simulink model "astron_hw_test_au50_64k"  (R2021a)
settings: Solver=VariableStepDiscrete  StartTime=0.0  StopTime=2048  RelTol=1e-3
undefined symbols (not defined in the file): d0, d1, d2, d3, FFT, sr, Wideband_FFT
libraries: xbsIndex_r4 x637, casper_library_misc x4, xps_library x1
(part 2 of 14)

== system astron_hw_test_au50_64k/bram_in0 ==
  addr : Inport
  data_in : Inport  Port=2
  we : Inport  Port=3
  Terminator : Terminator
  Terminator1 : Terminator
  Terminator2 : Terminator
  astron_hw_test_au50_64k_bram_in0_addr : xbsIndex_r4/Gateway Out  inherit_from_input=off  hdl_port=on  rows=1  columns=1  UseAsDAC=off  DACChannel='1'  interface=None  automatic_assignment=on  address_offset=hex2dec('00')  intf_name=''  intf_description=''  timing_constraint=None  locs_specified=off  LOCs={'A5','B9','A9','C1','A3','G6','E9','A6','A7','A8','B8','B1','B3','D9','B5','B4','B6','C2'}  io_standard={}  block_type=gatewayout
      settings: infoedit="Gateway out block.  Converts Xilinx fixed point inputs into ouputs of type Simulink integer, double, or fixed point.<P><P>Hardware notes:  In hardware these blocks become top level output ports or are discarded, depending on how they are configured."  sginterface={'Nallatech'=>{'xdspkit'=>{'non_memory_mapped_port'=>'uprev_Shared_BRAM_addr'}},'Xilinx'=>{'jtaghwcosim'=>{'non_memory_mapped_port'=>'uprev_Shared_BRAM_addr'},'xdspkit'=>{'non_memory_mapped_port'=>'uprev_Shared_BRAM_addr'}}}  xl_area=[0, 0, 0, 0, 0, 0, 0]
  astron_hw_test_au50_64k_bram_in0_data_in : xbsIndex_r4/Gateway Out  inherit_from_input=off  hdl_port=on  rows=1  columns=1  UseAsDAC=off  DACChannel='1'  interface=None  automatic_assignment=on  address_offset=hex2dec('00')  intf_name=''  intf_description=''  timing_constraint=None  locs_specified=off  LOCs={'B21','B22','A22','B23','B19','C19','A20','A21','A23','B24','A24','A25','E18','D18','C18','B18'}  io_standard={}  block_type=gatewayout
      settings: infoedit="Gateway out block.  Converts Xilinx fixed point inputs into ouputs of type Simulink integer, double, or fixed point.<P><P>Hardware notes:  In hardware these blocks become top level output ports or are discarded, depending on how they are configured."  sginterface={'Nallatech'=>{'xdspkit'=>{'non_memory_mapped_port'=>'uprev_Shared_BRAM_data_in'}},'Xilinx'=>{'jtaghwcosim'=>{'non_memory_mapped_port'=>'uprev_Shared_BRAM_data_in'},'xdspkit'=>{'non_memory_mapped_port'=>'uprev_Shared_BRAM_data_in'}}}  xl_area=[0, 0, 0, 0, 0, 0, 0]
  astron_hw_test_au50_64k_bram_in0_data_out : xbsIndex_r4/Gateway In  gui_display_data_type=Fixed-point  arith_type=Unsigned  n_bits=32  bin_pt=0  preci_type=Single  exp_width=8  frac_width=24  rows=1  columns=1  quantization=Truncate  overflow=Wrap  period=sample_rate  UseAsADC=off  ADCChannel='1'  interface=None  automatic_assignment=on  address_offset=hex2dec('00')  intf_name=''  intf_description=''  default_value=0  timing_constraint=None  locs_specified=off  LOCs={}  io_standard={}  inherit_from_input=off  hdl_port=on  dbl_ovrd=off  block_type=gatewayin
      settings: xl_area=[0, 0, 0, 0, 0, 0, 0]
  astron_hw_test_au50_64k_bram_in0_we : xbsIndex_r4/Gateway Out  inherit_from_input=off  hdl_port=on  rows=1  columns=1  UseAsDAC=off  DACChannel='1'  interface=None  automatic_assignment=on  address_offset=hex2dec('00')  intf_name=''  intf_description=''  timing_constraint=None  locs_specified=off  LOCs={'A14'}  io_standard={}  block_type=gatewayout
      settings: infoedit="Gateway out block.  Converts Xilinx fixed point inputs into ouputs of type Simulink integer, double, or fixed point.<P><P>Hardware notes:  In hardware these blocks become top level output ports or are discarded, depending on how they are configured."  xl_area=[0, 0, 0, 0, 0, 0, 0]
  calc_add : Subsystem  mask{data_width=32, addr_width=14, sample_rate=sample_rate}
      mask prompts: data_width "data width"; addr_width "address width"; sample_rate "sample rate"
  convert_addr : xbsIndex_r4/Convert  gui_display_data_type=Fixed-point  arith_type=Unsigned  n_bits=addr_width  bin_pt=0  float_type=Single  exp_bits=8  fraction_bits=24  quantization=Truncate  overflow=Wrap  en=off  latency=0  pipeline=off  dbl_ovrd=off  block_type=convert
      settings: xl_area=[0, 0, 0, 0, 0, 0, 0]
  convert_din1 : xbsIndex_r4/Convert  gui_display_data_type=Fixed-point  arith_type=Unsigned  n_bits=32  bin_pt=0  float_type=Single  exp_bits=8  fraction_bits=24  quantization=Truncate  overflow=Wrap  en=off  latency=0  pipeline=off  dbl_ovrd=off  block_type=convert
      settings: xl_area=[0, 0, 0, 0, 0, 0, 0]
  convert_we : xbsIndex_r4/Convert  gui_display_data_type=Fixed-point  arith_type=Unsigned  n_bits=1  bin_pt=0  float_type=Single  exp_bits=8  fraction_bits=24  quantization=Truncate  overflow=Wrap  en=off  latency=0  pipeline=off  dbl_ovrd=off  block_type=convert
      settings: xl_area=[0, 0, 0, 0, 0, 0, 0]
  munge_in : Subsystem  AncestorBlock=casper_library_flow_control/munge  mask(munge){divisions=1, div_size=32, order=[0], arith_type_out=Unsigned, bin_pt_out=0}
      mask prompts: divisions "Number of divisions"; div_size "Division size (bits)"; order "Division packing order"; arith_type_out "Output arithmetic type"; bin_pt_out "Output binary point"
      mask help: Splits an input bus into the specified number of divisions and then recombines them in the order specified (most significant division = 0,least = number divisions-1)
      mask init:
      | munge_init(gcb, ...
      |     'divisions', divisions, ...
      |     'div_size', div_size, ...
      |     'order', order, ...
      |     'arith_type_out', arith_type_out, ...
      |     'bin_pt_out', bin_pt_out);
      settings: AttributesFormatString=|
      | split:32
      | join:0
      | Unsigned [32,0]
      mask TypeOptions arith_type_out: Unsigned | Signed  (2's comp) | Floating-point
  munge_out : Subsystem  AncestorBlock=casper_library_flow_control/munge  mask(munge){divisions=1, div_size=32, order=[0], arith_type_out=Signed  (2's comp), bin_pt_out=0}
      mask prompts: divisions "Number of divisions"; div_size "Division size (bits)"; order "Division packing order"; arith_type_out "Output arithmetic type"; bin_pt_out "Output binary point"
      mask help: Splits an input bus into the specified number of divisions and then recombines them in the order specified (most significant division = 0,least = number divisions-1)
      mask init:
      | munge_init(gcb, ...
      |     'divisions', divisions, ...
      |     'div_size', div_size, ...
      |     'order', order, ...
      |     'arith_type_out', arith_type_out, ...
      |     'bin_pt_out', bin_pt_out);
      settings: AttributesFormatString=|
      | split:32
      | join:0
      | Signed  (2's comp) [32,0]
      mask TypeOptions arith_type_out: Unsigned | Signed  (2's comp) | Floating-point
  sim_mem : Subsystem  mask{arith_type=Signed  (2's comp), addr_width=14, data_width=32, data_bin_pt=0, init_vals=[1955   5372   -783    264   8673   2664   3057  -1583    502   -209  -3416  -8118   -695   2914  -2762  -1119  -2454   9156   1293  -1791   7946   -682  -6381  -1639  -3299  -1972   4876  -7418   8392   7738   1841  -6315   3917   6175   7083   2047   3941  -1371  -1683  -5922  -1392   1133   5033  -4748   -637   4947   1524  -7294  -1151    598   2939    694  -5379  -2771   7110 -11240   6719  -7297  -1947  -1257  -1047  10652  -8591  -4301  -4813    242   2319  -5536     54  -2316     44  -5035  -4892   -774   3868 -11427  -2970   5804   1082  -3502   4131  -2727   4137  -5631  -4745   5820   1584  -1336   1471   3152  -4149    207   2972   3505   -348  -2899   2818   3712  -2754  -5832    293   -548   -177    499   -115   -949  -5990    356   1812   4168   1094  -2711   3121   9110   4631  -1446   -611   -185  -6224  -7623   2980   5256    573   -721   7535  -2371   6280   1834  -3513  -3171   5430  -2617  -5379  -2004   1895  -5374  -4657   8059   -696  -8009   -392   3468   -741  -4248  -2142   6229   1080  -5263   2941   7567   1562    392    331  -2288   -850  -3689  -3788   -834   -495   3206   1798   -427   1349   2199   1760   3578   6351  -3080   1856   7720   5174  -4480    691  -1270   -965  -1827  -2279    789   7788  -3782   -204   2421   2427   3593    843    783    379   3234  -4266  10007  -1542  -5331  -3474  -3342    746   3673   3033   3588   2338    706   5614   4326   2572  -4419  -1161   -132   3707  -6818   5579   2728   3400  -1544   6105   2912   1907  -6007  -3653  -4264   2239  -5624  -4023   8559  -4168  -4103   6934  -1178  -3337   -386   2155   2151   6660  -2551  -1421  -1873   6722   3145  -8797   1273  -2565  -4488   2533  -2723  -4794    612   3317   -822   1310  -5199  -5455   4364   1455   8473   -163   5041 -11262   1818   1331  -1070   2800  -2280  -9404   3607  -1879  -3180    250   7444   5558  -4879   6913   6916  -7412  -2006  -1651   5554  -1733  -3584   1994    161    748   3913   5619   6382   -493   1474  -4417   -131  -7232  -6736  -4489  -3432  -3772   1085   1676   3615  -2928   -949  -2388    406    316  -3710  -2279  10859   5744   -234   4465   3318    351  -8376   3456   4924   1831   6284  -6721  -1230   -131  -6191  -1324   2438   4465   1240  -1945  -1100   2137  -7300   1759   6874  -2404  -1202  13311  -3786  -3231   -162   2575  -3936  -5274  -1656   7490   3000   2852  -2820   2433   2006  -2470  -1797   -562  -4165   6461  -1961   1271   3081   2229  -2189  -2454   2194   -963  -5197  -1235   5790  -2221   2148   -884   1526   4993 -12939  -4686   4539   -623   2170   2609   -302  -1091  -8231  -1744   4511   1350  -4644  -2187  -2325  -3974  -1395  -4542  -2217    937  -5029  -3543   -259  -1777    343  12537   4026  -3639  11402  -8467   9172  -1634    170   5494   3063  -7915   7245  -1426   2744  -2424   2974  -1244   -116   1945   2113   2591   5449   1931   -744   1325   1639   2812  -8436   1541   2860  -6413   7361  -8861   -750  -5957  -2950    778   5828   -643   4070  -4404   4301  -2747  -3510  -2107  -3373  -2842    239   6110   6919   9265   5964   3664   -550  -3103  -3159   1420   2494  -1468  -2931  -4676   3776   2828  -2781   4433  -1672  -1980    540    665  11327  -2200   3666  -1527   7426   -724  -7651  -3404   2220  -5721  -4925  -5276   5619  -2466   -307   4392   7830   1731  -8896  -2439   3110   3349  -7112  -7454   8450   3376   -647  -2091   5009   4298  -4269   -127   1593   3643  -3851   8300   1861   -140    757   1289   3866   1919    346  -5979    -32    725  -6926   3320  -2968   2732   -124   2491   2070  -1757  -6109  -7711  -1641   6611 -12060  -6128  -1216   1712  -2148  10157  -3305   3211   3381    782  -8059  -5771   -991   3862   5600  -7351    890  -6269   -676   9702  -8576  -1503   6527  -2901  -2235   3900   6327    999  -1480  -6646  -2544   4870  -3362   3523  -3643  -1996    176  -3592  -2266   6041  -4719  -2440   5604    446   1756  -4550  10810  -5848  -3044  -5127    204  -5769  -3243  -3026   5925   2337 ...(+110689 chars)], sample_rate=1, csp_latency=1}
      mask prompts: arith_type "Output Data Type"; addr_width "Address width"; data_width "Data width"; data_bin_pt "Data Binary Point"; init_vals "Initial values"; sample_rate "Sample rate"; csp_latency "Latency"
      mask init:
      | % set_param([gcb, '/data_to_xilinx'], 'arith_type', arith_type)
      | % set_param([gcb, '/data_to_xilinx'], 'n_bits', get_param(gcb, 'data_width'))
      mask TypeOptions arith_type: Unsigned | Signed  (2's comp)
      mask TypeOptions data_width: 8 | 16 | 32 | 64 | 128
  data_out : Outport  VectorParamsAs1DForOutWhenUnconnected=off
  wires:
  munge_out/1(dout) -> data_out/1
  sim_mem/1(data_out) -> astron_hw_test_au50_64k_bram_in0_data_out/1
  astron_hw_test_au50_64k_bram_in0_data_out/1 -> munge_out/1(din)
  convert_addr/1 -> astron_hw_test_au50_64k_bram_in0_addr/1
  convert_din1/1 -> astron_hw_test_au50_64k_bram_in0_data_in/1
  data_in/1 -> munge_in/1(din)
  calc_add/1(out) -> convert_addr/1
  astron_hw_test_au50_64k_bram_in0_we/1 -> Terminator2/1
  astron_hw_test_au50_64k_bram_in0_data_in/1 -> Terminator1/1
  astron_hw_test_au50_64k_bram_in0_addr/1 -> Terminator/1
  convert_we/1 -> astron_hw_test_au50_64k_bram_in0_we/1
  addr/1 -> sim_mem/1(addr), calc_add/1(in)
  we/1 -> sim_mem/3(we), convert_we/1
  munge_in/1(dout) -> sim_mem/2(data), convert_din1/1
